simulink model "mambo_realtime_simulator"  (R2022b)
settings: Solver=FixedStepAuto  StartTime=0.0  StopTime=inf  FixedStep=Ts  RelTol=1e-3
values from neighbouring files (symbols this model uses):
  K_gain_lin = lqr(A, B, Q_gain_lin, R_gain_lin)    [parrot_mambo_main.m]
  Ki_x = 0.04    [parrot_mambo_main.m]
  Ki_y = 0.04    [parrot_mambo_main.m]
  Ki_z = 0.023    [parrot_mambo_main.m]
  sat_z = 1    [parrot_mambo_main.m]
  Ts = 0.01    [parrot_mambo_main.m]
  x0 = -1.18    [parrot_mambo_main.m]
  y0 = -1.21    [parrot_mambo_main.m]
  z0 = 0.8    [parrot_mambo_main.m]
undefined symbols (not defined in the file or in its folder): rotation_matrix_from_Euler_123
libraries: cstblocks x15, simulink x3, etargetslib x2, dspnetwork x1, xpcutilitieslib x1, xpcrtudplib x1
settings Model: Creator=sanim  LastModifiedBy=phatdo
settings SolverCC: AlgebraicLoopSolver=TrustRegion
settings DataIOCC: ReturnWorkspaceOutputs=off
settings DebuggingCC: ParameterOverflowMsg=none  UnconnectedInputMsg=warning  UnconnectedOutputMsg=warning  UnconnectedLineMsg=warning  SFMachineParentedDataDiag=warning  ArithmeticOperatorsInVariantConditions=warning
settings ModelReferenceCC: EnableRefExpFcnMdlSchedulingChecks=on
settings SFSimCC: CustomCodeUndefinedFunction=UseInterfaceOnly
settings RTWCC: Description=Simulink Desktop Real-Time  SystemTargetFile=sldrt.tlc  TemplateMakefile=sldrt.tmf  RTWCompilerOptimization=on
settings CodeAppCC: MaxIdLength=95  StateflowObjectComments=on
settings SimulinkDesktopRealTimeCC: TargetPreCompLibLocation=C:\Program Files\MATLAB\R2018b\toolbox\sldrt\lib\win64

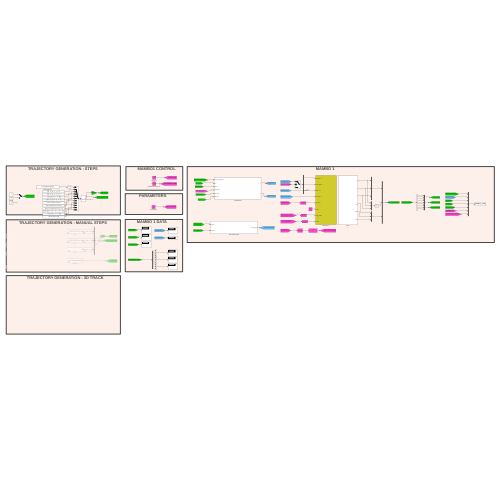
[thumbnail: Simulink's stored preview of the top-level diagram]
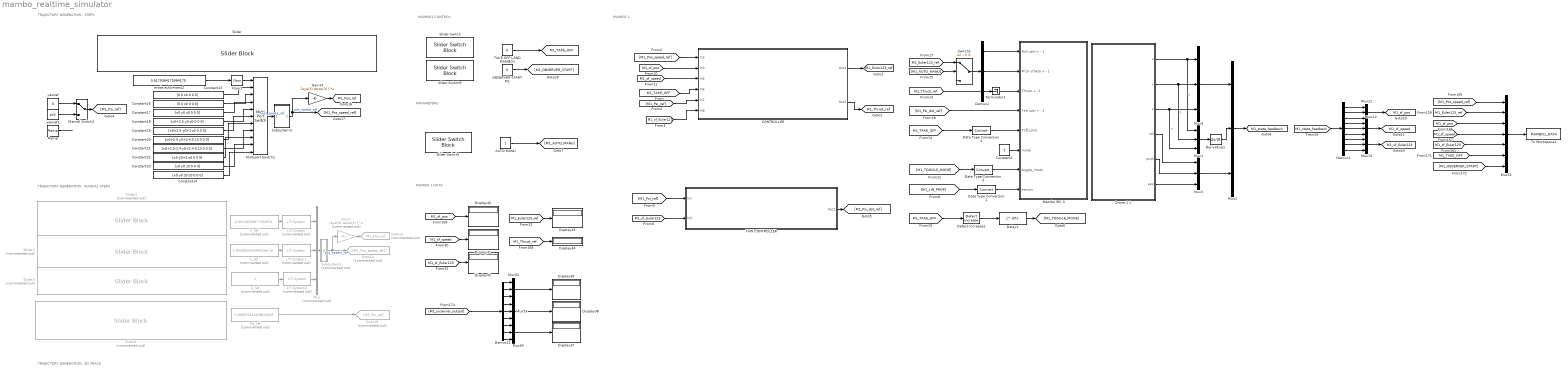
== system mambo_realtime_simulator ==
  note: MAMBO1 CONTROL
  note: MAMBO 1
  note: MAMBO 1 DATA
  note: TRAJECTORY GENERATION : STEPS
  note: PARAMETERS
  note: TRAJECTORY GENERATION : 3D TRACK
  note: TRAJECTORY GENERATION : MANUAL STEPS
  AUTO MANU : Constant
  CONTROLLER : Subsystem
  Constant1 : Constant  Value=2  OutDataTypeStr=uint8
  Constant14 : Constant  Value=[x0 y0 z0-z0 0 0 0]
  Constant15 : Constant  Value=[0 0 z0 0 0 0]
  Constant16 : Constant  Value=[0 0 z0 0 0 0]
  Constant17 : Constant  Value=[x0 y0 z0 0 0 0]
  Constant18 : Constant  Value=[x0+2.5 y0 z0 0 0 0]
  Constant19 : Constant  Value=[x0+2.5 y0+1 z0 0 0 0]
  Constant20 : Constant  Value=[x0+2.5 y0+2.4 0.13 0 0 0]
  Constant21 : Constant  Value=[x0+2.5-2.4 y0+2.4 0.13 0 0 0]
  Constant22 : Constant  Value=[x0 y0+2 z0 0 0 0]
  Constant23 : Constant  Value=[x0 y0 z0 0 0 0]
  Data Type Conversion1 : DataTypeConversion  SaturateOnIntegerOverflow=off  RndMeth=Floor
  Data Type Conversion3 : DataTypeConversion  SaturateOnIntegerOverflow=off  RndMeth=Floor
  Data Type Conversion4 : DataTypeConversion  SaturateOnIntegerOverflow=off  RndMeth=Floor
  Delay1 : Delay  DelayLength=3/Ts
  Demux1 : Demux  Outputs=3
  Demux11 : Demux  Outputs=9
  Demux3 : Demux  Outputs=9
  Derivative1 : Derivative  CoefficientInTFapproximation=4*Ts
  Detect Increase2 : simulink/Logic and Bit Operations/Detect Increase  vinit=0.0  OutDataTypeStr=uint8
  Display{37..44} (8 alike) : Display
  Drone 1 1 : Subsystem
  Floor1 : Rounding
  Gain1 : Gain  Commented=on  Gain=[eye(3) zeros(3) ]  Multiplication=Matrix(K*u) (u vector)
  Gain14 : Gain  Gain=[eye(3) zeros(3) ]  Multiplication=Matrix(K*u) (u vector)
  Goto13 : Goto  Commented=on  GotoTag=M1_Pos_ref  TagVisibility=global
  Goto14 : Goto  Commented=on  GotoTag=M1_Pos_speed_ref
  Goto15 : Goto  Commented=on  GotoTag=M1_Psi_ref
  LTI System : cstblocks/LTI System  Commented=on  sys=tf(1,[0.35 1.2 1])  IC=[]
  LTI System1 : cstblocks/LTI System  Commented=on  sys=tf(1,[0.35 1.2 1])  IC=[]
  LTI System2 : cstblocks/LTI System  Commented=on  sys=tf(1,[0.35 1.2 1])  IC=[]
  Mambo IRC 3 : Subsystem
  Manual Switch2 : ManualSwitch
  Multiport Switch1 : MultiPortSwitch  DataPortOrder=Zero-based contiguous  Inputs=10  zeroidx=on  SaturateOnIntegerOverflow=off  InputSameDT=off
  Mux : Mux  Commented=on  Inputs=3
  Mux{1..4,11..13,52..54} (10 alike) : Mux  Inputs=3
  Mux51 : Mux  Inputs=7
  OBSERVER START M1 : Constant  Value=0
  Psi_ref : Constant  Commented=on  Value=0.009876543209876409  OutDataTypeStr=double
  Ramp : simulink/Sources/Ramp  slope=1  start=20  InitialOutput=0
  Slider : SliderBlock  ScaleMax=10  TickInterval=1
  Slider Switch : SliderSwitchBlock
      settings: Values={{'Off', 'On'}, [0 1]}
  Slider Switch1 : SliderSwitchBlock
      settings: Values={{'Off', 'On'}, [0 1]}
  Slider Switch9 : SliderSwitchBlock
      settings: Values={{'Off', 'On'}, [0 1]}
  Slider1 : SliderBlock  Commented=on  ScaleMin=-1.6000000000000001  ScaleMax=1.6000000000000001  TickInterval=0.10000000000000001
  Slider2 : SliderBlock  Commented=on  ScaleMin=-1.6000000000000001  ScaleMax=1.6000000000000001  TickInterval=0.10000000000000001
  Slider3 : SliderBlock  Commented=on  ScaleMax=2  TickInterval=0.10000000000000001
  Slider4 : SliderBlock  Commented=on  ScaleMin=-4  ScaleMax=4  TickInterval=0.10000000000000001
  Subsystem1 : Subsystem  Commented=on
  Subsystem3 : Subsystem
  Switch1 : Switch  Criteria=u2 ~= 0  SaturateOnIntegerOverflow=off  InputSameDT=off
  TAKE OFF LAND MAMBO1 : Constant  Value=0
  Terminator1 : Terminator
  To Workspace1 : ToWorkspace  VariableName=MAMBO1_DATA  SaveFormat=Timeseries  SampleTime=-1
  X_ref : Constant  Commented=on  Value=-0.00140350877192974  OutDataTypeStr=double
  YAW CONTROLLER : Subsystem
  Y_ref : Constant  Commented=on  Value=1.942890293094024e-16  OutDataTypeStr=double
  Z_ref : Constant  Commented=on  OutDataTypeStr=double
  mode auto/manu2 : Constant  Value=0.9175084175084175  OutDataTypeStr=double
  yawref : Constant  Value=0  OutDataTypeStr=double
  yawref1 : Constant  Value=pi/2  OutDataTypeStr=double
  tag scope: M1_Euler123_ref=global, M1_Pos_ref=global, M1_TAKE_OFF=global, M1_Thrust_ref=global, M1_sf_Euler123=global, M1_sf_pos=global, M1_sf_speed=global, M1_state_feedback=global
  wires:
  [M1_state_feedback] -> Demux3/1
  Demux3/7 -> Mux13/1
  Mux12/1 -> [M1_sf_speed]
  Demux3/3 -> Mux11/3
  Demux3/6 -> Mux12/3
  Mux11/1 -> [M1_sf_pos]
  Demux3/1 -> Mux11/1
  Demux3/5 -> Mux12/2
  Mux13/1 -> [M1_sf_Euler123]
  Demux3/4 -> Mux12/1
  Demux3/8 -> Mux13/2
  Demux3/2 -> Mux11/2
  Demux3/9 -> Mux13/3
  Gain14/1 -> [M1_Pos_ref]
  TAKE OFF LAND MAMBO1/1 -> [M1_TAKE_OFF]
  AUTO MANU/1 -> [M1_AUTO_MANU]
  [M1_Psi_ref] -> YAW CONTROLLER/1(In1)
  [M1_sf_Euler123] -> YAW CONTROLLER/2(In2)
  YAW CONTROLLER/1(Out1) -> [M1_Psi_dot_ref]
  yawref/1 -> Manual Switch2/1
  Manual Switch2/1 -> [M1_Psi_ref]
  Ramp/1 -> ?
  Mux51/1 -> To Workspace1/1
  [M1_Euler123_ref] -> Mux51/2
  Demux11/6 -> Mux53/3
  [M1_sf_speed] -> Display41/1
  [M1_sf_pos] -> Display40/1
  Demux11/1 -> Mux52/1
  Demux11/5 -> Mux53/2
  [M1_Pos_speed_ref] -> Mux51/1
  Demux11/3 -> Mux52/3
  [M1_Euler123_ref] -> Display43/1
  Mux54/1 -> Display37/1
  Demux11/8 -> Mux54/2
  Demux11/2 -> Mux52/2
  Demux11/7 -> Mux54/1
  [M1_ovserver_output] -> Demux11/1
  Demux11/4 -> Mux53/1
  [M1_OBSERVER_START] -> Mux51/7
  Mux52/1 -> Display39/1
  [M1_sf_speed] -> Mux51/4
  Demux11/9 -> Mux54/3
  [M1_sf_Euler123] -> Display42/1
  [M1_sf_pos] -> Mux51/3
  [M1_sf_Euler123] -> Mux51/5
  [M1_Thrust_ref] -> Display44/1
  Mux53/1 -> Display38/1
  OBSERVER START M1/1 -> [M1_OBSERVER_START]
  yawref1/1 -> Manual Switch2/2
  Subsystem3/1(Out1) -> [M1_Pos_speed_ref], Gain14/1  "pos_speed_ref"
  Data Type Conversion3/1 -> Mambo IRC 3/7(toggle_mode)
  [M1_TOGGLE_MODE] -> Data Type Conversion3/1
  Data Type Conversion4/1 -> Mambo IRC 3/5(Toff_Land)
  Switch1/1 -> Demux1/1
  Detect Increase2/1 -> Delay1/1
  [M1_LIN_PROP] -> Data Type Conversion1/1
  [M1_TAKE_OFF] -> Data Type Conversion4/1
  Delay1/1 -> [M1_TOGGLE_MODE]
  [M1_AUTO_MANU] -> Switch1/2
  [M1_TAKE_OFF] -> Detect Increase2/1
  Demux1/1 -> Mambo IRC 3/1(Roll uphi + - 1)
  [M1_Thrust_ref] -> Mambo IRC 3/3(Thrust + - 1)
  Constant1/1 -> Mambo IRC 3/6(mode)
  [M1_Psi_dot_ref] -> Mambo IRC 3/4(Yaw upsi + - 1)
  Derivative1/1 -> Mux2/2
  Mux2/1 -> [M1_state_feedback]
  [M1_Euler123_ref] -> Switch1/1
  Drone 1 1/2(y) -> Mux1/2, Mux4/2  "y"
  Mux1/1 -> Derivative1/1
  Demux1/3 -> Terminator1/1
  Demux1/2 -> Mambo IRC 3/2(Pitch utheta + - 1)
  Drone 1 1/4(roll) -> Mux3/1
  Mux4/1 -> Mux2/1
  Drone 1 1/5(pitch) -> Mux3/2
  Drone 1 1/1(x) -> Mux1/1, Mux4/1  "x"
  Mux3/1 -> Mux2/3
  Drone 1 1/6(yaw) -> Mux3/3
  Drone 1 1/3(z) -> Mux1/3, Mux4/3  "z"
  Subsystem1/1(Out1) -> Gain1/1, Goto14/1  "pos_speed_ref"
  Gain1/1 -> Goto13/1
  Y_ref/1 -> LTI System1/1
  Z_ref/1 -> LTI System2/1
  X_ref/1 -> LTI System/1
  Mux/1 -> Subsystem1/1(In1)
  Psi_ref/1 -> Goto15/1
  LTI System/1 -> Mux/1
  LTI System1/1 -> Mux/2
  LTI System2/1 -> Mux/3
  Data Type Conversion1/1 -> Mambo IRC 3/8(cannon)
  [M1_TAKE_OFF] -> Mux51/6
  CONTROLLER/1(Out1) -> [M1_Euler123_ref]
  CONTROLLER/2(Out2) -> [M1_Thrust_ref]
  [M1_Psi_ref] -> CONTROLLER/5(In7)
  [M1_sf_Euler123] -> CONTROLLER/6(In8)
  [M1_TAKE_OFF] -> CONTROLLER/4(In6)
  [M1_sf_pos] -> CONTROLLER/2(In3)
  [M1_sf_speed] -> CONTROLLER/3(In5)
  [M1_Pos_speed_ref] -> CONTROLLER/1(In2)
  Constant15/1 -> Multiport Switch1/2
  Constant17/1 -> Multiport Switch1/4
  Constant14/1 -> Multiport Switch1/11
  Constant21/1 -> Multiport Switch1/8
  Constant16/1 -> Multiport Switch1/3
  Constant20/1 -> Multiport Switch1/7
  Constant22/1 -> Multiport Switch1/9
  Constant23/1 -> Multiport Switch1/10
  Floor1/1 -> Multiport Switch1/1
  mode auto/manu2/1 -> Floor1/1
  Constant18/1 -> Multiport Switch1/5
  Constant19/1 -> Multiport Switch1/6
  Multiport Switch1/1 -> Subsystem3/1(In1)  "pos_speed_ref"

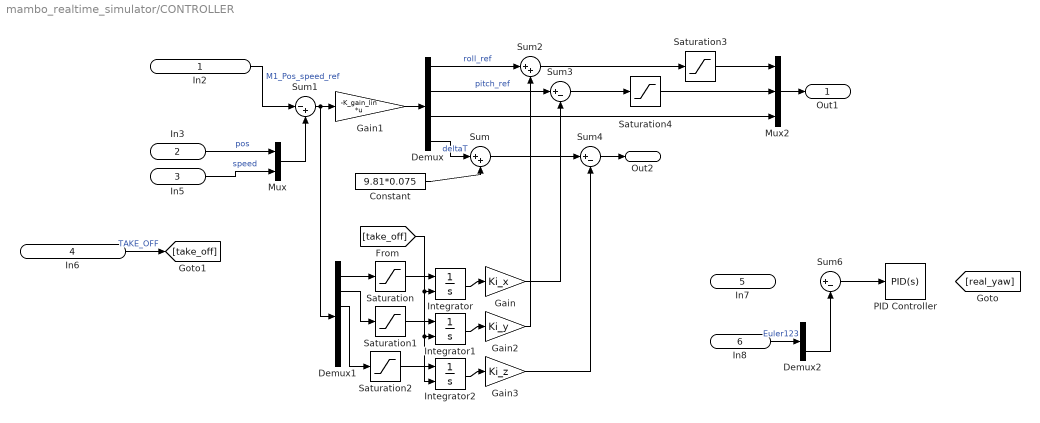
== system mambo_realtime_simulator/CONTROLLER ==
  In2 : Inport
  In3 : Inport  Port=2
  In5 : Inport  Port=3
  In6 : Inport  Port=4
  In7 : Inport  Port=5
  In8 : Inport  Port=6
  Constant : Constant  Value=9.81*0.075
  Demux : Demux
  Demux1 : Demux  Outputs=6
  Demux2 : Demux  Outputs=3
  Gain : Gain  Gain=Ki_x
  Gain1 : Gain  Gain=-K_gain_lin  Multiplication=Matrix(K*u) (u vector)
  Gain2 : Gain  Gain=Ki_y
  Gain3 : Gain  Gain=Ki_z
  Integrator : Integrator  ExternalReset=rising
  Integrator1 : Integrator  ExternalReset=rising
  Integrator2 : Integrator  ExternalReset=rising
  Mux : Mux  Inputs=2
  Mux2 : Mux  Inputs=3
  PID Controller : simulink/Continuous/PID Controller  Controller=PID  Form=Parallel  TimeDomain=Continuous-time  SampleTime=-1  IntegratorMethod=Forward Euler  FilterMethod=Forward Euler  ControllerParametersSource=internal  P=1.9  I=4.5  D=0.05  UseFilter=on  N=8.8  TunerSelectOption=Transfer Function Based (PID Tuner App)  InitialConditionSource=internal  InitialConditionForIntegrator=0  InitialConditionForFilter=0  DifferentiatorICPrevScaledInput=0  ExternalReset=none  TrackingMode=off  Kt=1  LimitOutput=off  UpperSaturationLimit=inf  LowerSaturationLimit=-inf  LinearizeAsGain=on  AntiWindupMode=none  Kb=1  POutMin=[]  POutMax=[]  IOutMin=[]  IOutMax=[]  DOutMin=[]  DOutMax=[]  NOutMin=[]  NOutMax=[]  SumOutMin=[]  SumOutMax=[]  SaturationOutMin=[]  SaturationOutMax=[]  PParamMin=[]  PParamMax=[]  IParamMin=[]  IParamMax=[]  DParamMin=[]  DParamMax=[]  NParamMin=[]  NParamMax=[]  KbParamMin=[]  KbParamMax=[]  KtParamMin=[]  KtParamMax=[]  KbOutMin=[]  KbOutMax=[]  KtOutMin=[]  KtOutMax=[]  IntegratorOutMin=[]  IntegratorOutMax=[]  FilterOutMin=[]  FilterOutMax=[]  SumI1OutMin=[]  SumI1OutMax=[]  SumI2OutMin=[]  SumI2OutMax=[]  SumI3OutMin=[]  SumI3OutMax=[]  SumI4OutMin=[]  SumI4OutMax=[]  SumDOutMin=[]  SumDOutMax=[]  DifferentiatorOutMin=[]  DifferentiatorOutMax=[]  FilterDiffOutCoefMin=[]  FilterDiffOutCoefMax=[]  ReciprocalOutMin=[]  ReciprocalOutMax=[]  SumDenOutMin=[]  SumDenOutMax=[]  SumNumOutMin=[]  SumNumOutMax=[]  DivideOutMin=[]  DivideOutMax=[]  IntegratorContinuousStateAttributes=''  IntegratorStateMustResolveToSignalObject=off  IntegratorRTWStateStorageClass=Auto  FilterContinuousStateAttributes=''  FilterStateMustResolveToSignalObject=off  FilterRTWStateStorageClass=Auto  ParallelPVariant=InternalParameters  IdealPVariant=Disabled  IVariant=InternalParameters  DVariant=InternalParameters  IntegratorVariant=Continuous  SatVariant=Disabled  AWVariant=Passthrough  PCopyVariant=Disabled  TRVariant=Disabled  FdbkBlocksVariant=Forward  IdealPFdbkVariant=Disabled  SatFdbkVariant=Disabled  DerivativeFilterVariant=ContFilter  NVariant=InternalParameters  NCopyVariant=Disabled  FilterICVariant=InternalICsFilter  IntegratorICVariant=InternalICs  ExternalResetVariant=Disabled  TRSumVariant=Passthrough  SumFdbkVariant=Disabled  SumVariant=Sum_PID
  Saturation : Saturate  UpperLimit=0.02  LowerLimit=-0.02
  Saturation1 : Saturate  UpperLimit=0.02  LowerLimit=-0.02
  Saturation2 : Saturate  UpperLimit=sat_z  LowerLimit=-sat_z
  Saturation3 : Saturate  UpperLimit=0.1  LowerLimit=-0.1
  Saturation4 : Saturate  UpperLimit=0.1  LowerLimit=-0.1
  Sum : Sum  Inputs=|++
  Sum1 : Sum  Inputs=|-+
  Sum2 : Sum  Inputs=|++
  Sum3 : Sum  Inputs=|+-
  Sum4 : Sum  Inputs=|+-
  Sum6 : Sum  Inputs=|+-
  Out1 : Outport
  Out2 : Outport  Port=2
  wires:
  Sum1/1 -> Demux1/1, Gain1/1
  In2/1 -> Sum1/1  "M1_Pos_speed_ref"
  Mux/1 -> Sum1/2
  Gain1/1 -> Demux/1
  In5/1 -> Mux/2  "speed"
  Mux2/1 -> Out1/1
  Constant/1 -> Sum/2
  Demux/4 -> Sum/1  "deltaT"
  In3/1 -> Mux/1  "pos"
  Demux1/3 -> Saturation2/1
  Demux1/1 -> Saturation/1
  Demux/1 -> Sum2/1  "roll_ref"
  Sum2/1 -> Saturation3/1
  Demux/2 -> Sum3/1  "pitch_ref"
  Sum3/1 -> Saturation4/1
  Sum4/1 -> Out2/1
  Sum/1 -> Sum4/1
  Integrator2/1 -> Gain3/1
  Gain/1 -> Sum3/2
  Gain2/1 -> Sum2/2
  Integrator/1 -> Gain/1
  Integrator1/1 -> Gain2/1
  Gain3/1 -> Sum4/2
  Saturation/1 -> Integrator/1
  Saturation1/1 -> Integrator1/1
  Demux1/2 -> Saturation1/1
  Demux/3 -> Mux2/3
  In8/1 -> Demux2/1  "Euler123"
  Sum6/1 -> PID Controller/1
  Demux2/3 -> Sum6/2
  Saturation2/1 -> Integrator2/1
  Saturation3/1 -> Mux2/1
  Saturation4/1 -> Mux2/2
  In6/1 -> [take_off]  "TAKE_OFF"
  [take_off] -> Integrator2/2, Integrator1/2, Integrator/2

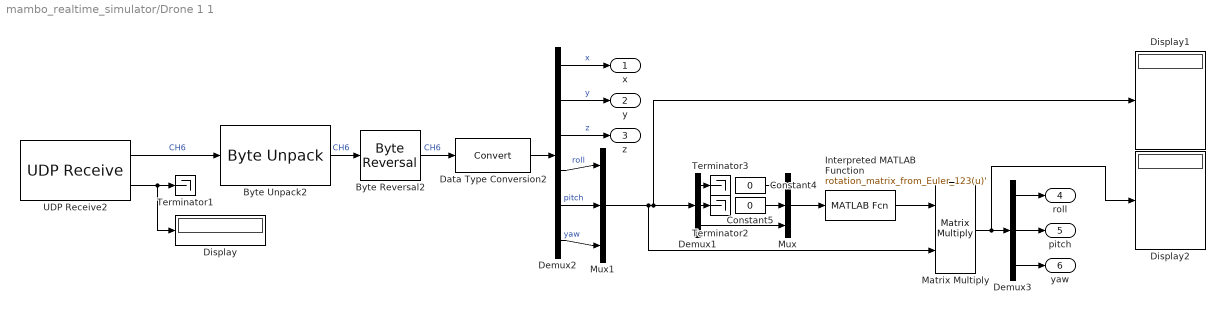
== system mambo_realtime_simulator/Drone 1 1 ==
  Byte Reversal2 : etargetslib/Byte Reversal  numInp=1
  Byte Unpack2 : etargetslib/Byte Unpack  dimensions={[6,1]}  datatypes={'single'}  byteAlign=1
  Constant4 : Constant  Value=0
  Constant5 : Constant  Value=0
  Data Type Conversion2 : DataTypeConversion  SaturateOnIntegerOverflow=off  RndMeth=Floor
  Demux1 : Demux  Outputs=3
  Demux2 : Demux  Outputs=6
  Demux3 : Demux  Outputs=3
  Display : Display
  Display1 : Display
  Display2 : Display
  Interpreted MATLAB Function : MATLABFcn  MATLABFcn=rotation_matrix_from_Euler_123(u)'  OutputDimensions=[3, 3]  Output1D=off
  Matrix Multiply : Product  Multiplication=Matrix(*)
  Mux : Mux  Inputs=3
  Mux1 : Mux  Inputs=3
  Terminator1 : Terminator
  Terminator2 : Terminator
  Terminator3 : Terminator
  UDP Receive2 : dspnetwork/UDP Receive  localURL='0.0.0.0'  localPort=38001  remoteURL='192.168.0.50'  remotePort=-1  recvBufferSize=24  dims=24  signalDatatype=uint8  isVarSize=off  showBlockingTime=on  blockingTime=Ts  sampletime=Ts  blockPlatform=HOST
  x : Outport
  y : Outport  Port=2
  z : Outport  Port=3
  roll : Outport  Port=4
  pitch : Outport  Port=5
  yaw : Outport  Port=6
  wires:
  Demux2/3 -> z/1  "z"
  UDP Receive2/1 -> Byte Unpack2/1  "CH6"
  Byte Unpack2/1 -> Byte Reversal2/1  "CH6"
  Demux2/2 -> y/1  "y"
  Byte Reversal2/1 -> Data Type Conversion2/1  "CH6"
  Data Type Conversion2/1 -> Demux2/1
  Demux2/1 -> x/1  "x"
  UDP Receive2/2 -> Display/1, Terminator1/1
  Matrix Multiply/1 -> Display2/1, Demux3/1
  Demux1/2 -> Terminator2/1
  Demux1/3 -> Mux/3
  Constant4/1 -> Mux/1
  Interpreted MATLAB Function/1 -> Matrix Multiply/1
  Demux1/1 -> Terminator3/1
  Constant5/1 -> Mux/2
  Mux/1 -> Interpreted MATLAB Function/1
  Mux1/1 -> Matrix Multiply/2, Display1/1, Demux1/1
  Demux2/4 -> Mux1/1  "roll"
  Demux2/5 -> Mux1/2  "pitch"
  Demux2/6 -> Mux1/3  "yaw"
  Demux3/2 -> pitch/1
  Demux3/1 -> roll/1
  Demux3/3 -> yaw/1

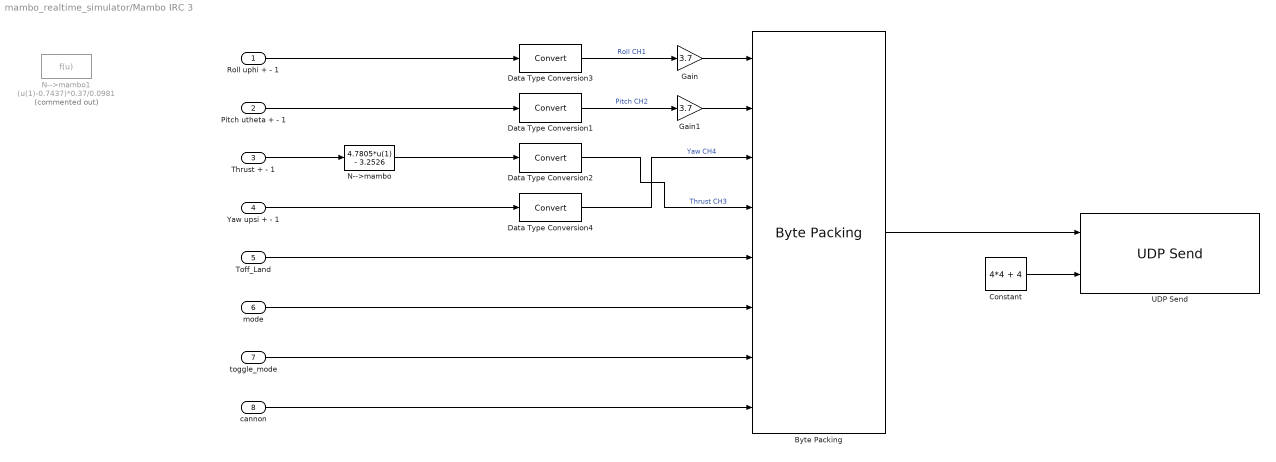
== system mambo_realtime_simulator/Mambo IRC 3 ==
  Roll uphi + - 1 : Inport
  Pitch utheta + - 1 : Inport  Port=2
  Thrust + - 1 : Inport  Port=3
  Yaw upsi + - 1 : Inport  Port=4
  Toff_Land : Inport  Port=5
  mode : Inport  Port=6
  toggle_mode : Inport  Port=7
  cannon : Inport  Port=8
  "Byte Packing " : xpcutilitieslib/Byte Packing   MaskPackedDataType=uint8  MaskUnpackedDataTypes={'single','single','single','single','uint8','uint8','uint8','uint8'}  MaskAlignment=1
  Constant : Constant  Value=4*4 + 4  SampleTime=Ts
  Data Type Conversion{1..4} (4 alike) : DataTypeConversion  SaturateOnIntegerOverflow=off  RndMeth=Floor
  Gain : Gain  Gain=3.7
  Gain1 : Gain  Gain=3.7
  N-->mambo : Fcn  Expr="4.7805*u(1)  - 3.2526"
  N-->mambo1 : Fcn  Commented=on  Expr=(u(1)-0.7437)*0.37/0.0981
  UDP Send : xpcrtudplib/UDP Send  ipAddressVal=Use host-target connection  localPort=-1  toAddress=192.168.0.50  toPort=38101  sampleTime=Ts
  wires:
  Gain1/1 -> "Byte Packing "/2
  Gain/1 -> "Byte Packing "/1
  Data Type Conversion2/1 -> "Byte Packing "/4  "Thrust CH3"
  Data Type Conversion4/1 -> "Byte Packing "/3  "Yaw CH4"
  N-->mambo/1 -> Data Type Conversion2/1
  Roll uphi + - 1/1 -> Data Type Conversion3/1
  Pitch utheta + - 1/1 -> Data Type Conversion1/1
  Thrust + - 1/1 -> N-->mambo/1
  Yaw upsi + - 1/1 -> Data Type Conversion4/1
  Data Type Conversion1/1 -> Gain1/1  "Pitch CH2"
  Data Type Conversion3/1 -> Gain/1  "Roll CH1"
  mode/1 -> "Byte Packing "/6
  cannon/1 -> "Byte Packing "/8
  Toff_Land/1 -> "Byte Packing "/5
  toggle_mode/1 -> "Byte Packing "/7
  Constant/1 -> UDP Send/2
  "Byte Packing "/1 -> UDP Send/1

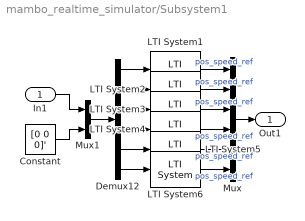
== system mambo_realtime_simulator/Subsystem1 ==
  In1 : Inport
  Constant : Constant  Value=[0 0 0]'
  Demux12 : Demux  Outputs=6
  LTI System{1..6} (6 alike) : cstblocks/LTI System  sys=tf(1,[0.01 1])  IC=[]
  Mux : Mux  Inputs=6
  Mux1 : Mux  Inputs=2
  Out1 : Outport
  wires:
  LTI System6/1 -> Mux/6  "pos_speed_ref"
  LTI System4/1 -> Mux/4  "pos_speed_ref"
  Demux12/4 -> LTI System4/1
  LTI System3/1 -> Mux/3  "pos_speed_ref"
  Demux12/6 -> LTI System6/1
  LTI System5/1 -> Mux/5  "pos_speed_ref"
  Demux12/5 -> LTI System5/1
  LTI System1/1 -> Mux/1  "pos_speed_ref"
  Demux12/3 -> LTI System3/1
  Mux/1 -> Out1/1
  Demux12/2 -> LTI System2/1
  LTI System2/1 -> Mux/2  "pos_speed_ref"
  Demux12/1 -> LTI System1/1
  In1/1 -> Mux1/1
  Constant/1 -> Mux1/2
  Mux1/1 -> Demux12/1

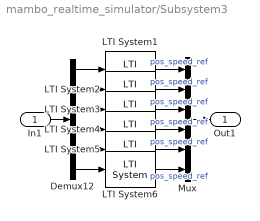
== system mambo_realtime_simulator/Subsystem3 ==
  In1 : Inport
  Demux12 : Demux  Outputs=6
  LTI System{1..6} (6 alike) : cstblocks/LTI System  sys=tf(1,[0.01 1])  IC=[]
  Mux : Mux  Inputs=6
  Out1 : Outport
  wires:
  In1/1 -> Demux12/1
  Demux12/1 -> LTI System1/1
  LTI System2/1 -> Mux/2  "pos_speed_ref"
  Demux12/2 -> LTI System2/1
  Mux/1 -> Out1/1
  Demux12/3 -> LTI System3/1
  LTI System1/1 -> Mux/1  "pos_speed_ref"
  Demux12/5 -> LTI System5/1
  LTI System5/1 -> Mux/5  "pos_speed_ref"
  Demux12/6 -> LTI System6/1
  LTI System3/1 -> Mux/3  "pos_speed_ref"
  Demux12/4 -> LTI System4/1
  LTI System4/1 -> Mux/4  "pos_speed_ref"
  LTI System6/1 -> Mux/6  "pos_speed_ref"

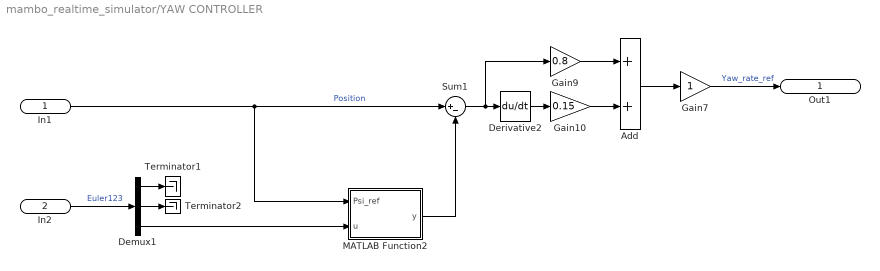
== system mambo_realtime_simulator/YAW CONTROLLER ==
  In1 : Inport
  In2 : Inport  Port=2
  Add : Sum
  Demux1 : Demux  Outputs=3
  Derivative2 : Derivative  CoefficientInTFapproximation=4*Ts
  Gain10 : Gain  Gain=0.15
  Gain7 : Gain
  Gain9 : Gain  Gain=0.8
  MATLAB Function2 : MATLAB Function  TreatAsAtomicUnit=on
  Sum1 : Sum  Inputs=|+-
  Terminator1 : Terminator
  Terminator2 : Terminator
  Out1 : Outport
  wires:
  Sum1/1 -> Gain9/1, Derivative2/1
  Gain9/1 -> Add/1
  Gain10/1 -> Add/2
  Add/1 -> Gain7/1
  Derivative2/1 -> Gain10/1
  Demux1/2 -> Terminator2/1
  In1/1 -> MATLAB Function2/1(Psi_ref), Sum1/1  "Position"
  In2/1 -> Demux1/1  "Euler123"
  Demux1/1 -> Terminator1/1
  Gain7/1 -> Out1/1  "Yaw_rate_ref"
  Demux1/3 -> MATLAB Function2/2(u)
  MATLAB Function2/1(y) -> Sum1/2

== matlab function mambo_realtime_simulator/YAW CONTROLLER/MATLAB Function2 ==
  data: Psi_ref input; u input; y output
function y = fcn(Psi_ref, u)
    y = u ;
    if Psi_ref > 0 && u < 0
        y = -u ;
    end
    
    if Psi_ref < 0 && u > 0
        y = -u ;
    end

end
